simulink model "PMSM_SquareWave"  (R2021b)
settings: Solver=VariableStepAuto  StartTime=0.0  StopTime=500e-6  MaxStep=5e-8  RelTol=1e-5
InitFcn:
  | % Loading the measurement data
  | load('MeasurementData.mat', 'PM')
libraries: SLNS x2, simulink x2, simulink_extras x1
settings Model: Creator=Szalay  LastModifiedBy=Szalay
settings SolverCC: AlgebraicLoopSolver=TrustRegion
settings DebuggingCC: SFMachineParentedDataDiag=warning

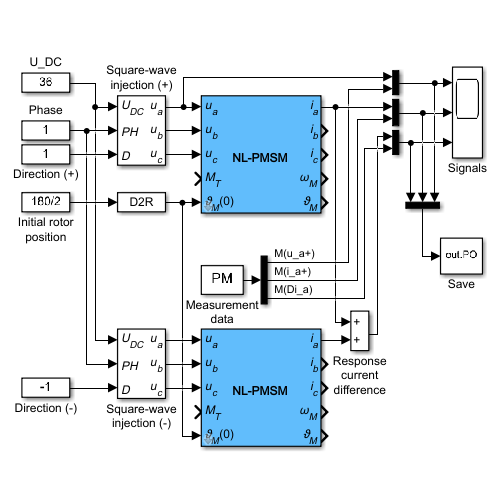
[thumbnail: Simulink's stored preview of the top-level diagram]
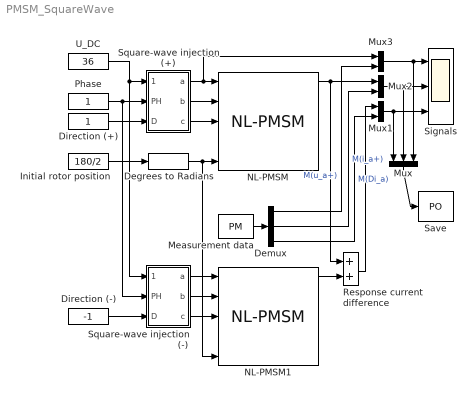
== system PMSM_SquareWave ==
  Degrees to Radians : simulink_extras/Transformations/Degrees to Radians
  Demux : Demux  Outputs=3
  Direction (+) : Constant
  Direction (-) : Constant  Value=-1
  Initial rotor position : Constant  Value=180/2
  Measurement data : FromWorkspace  VariableName=PM  SampleTime=-1  Interpolate=off  OutputAfterFinalValue=Setting to zero
  Mux : Mux  Inputs=3
  Mux1 : Mux  Inputs=2
  Mux2 : Mux  Inputs=2
  Mux3 : Mux  Inputs=2
  NL-PMSM : SLNS/Electric machines/NL-PMSM  varZp=2  varRs=0.654  varF_PM=24.83  varLd=145  varLq=188  varG_0=0.16  varB=6.329e-3  varJ=200  i_d0=0  i_q0=0
  NL-PMSM1 : SLNS/Electric machines/NL-PMSM  varZp=2  varRs=0.654  varF_PM=24.83  varLd=145  varLq=188  varG_0=0.16  varB=6.329e-3  varJ=200  i_d0=0  i_q0=0
  Phase : Constant
  Response current difference : Sum
  Save : ToWorkspace  VariableName=PO  SampleTime=1/240000
  Signals : Scope  NumInputPorts=3
  Square-wave injection (+) : Subsystem
      mask Display:
      | port_label('input', 1, '\itU_{DC}', 'texmode', 'on');
      | port_label('input', 2, '\itPH', 'texmode', 'on');
      | port_label('input', 3, '\itD', 'texmode', 'on');
      | 
      | port_label('output', 1, '\itu_a', 'texmode', 'on');
      | port_label('output', 2, '\itu_b', 'texmode', 'on');
      | port_label('output', 3, '\itu_c', 'texmode', 'on');
  Square-wave injection (-) : Subsystem
      mask Display:
      | port_label('input', 1, '\itU_{DC}', 'texmode', 'on');
      | port_label('input', 2, '\itPH', 'texmode', 'on');
      | port_label('input', 3, '\itD', 'texmode', 'on');
      | 
      | port_label('output', 1, '\itu_a', 'texmode', 'on');
      | port_label('output', 2, '\itu_b', 'texmode', 'on');
      | port_label('output', 3, '\itu_c', 'texmode', 'on');
  U_DC : Constant  Value=36
  wires:
  Initial rotor position/1 -> Degrees to Radians/1
  Square-wave injection (+)/1(a) -> NL-PMSM/1, Mux3/1
  Square-wave injection (+)/2(b) -> NL-PMSM/2
  Measurement data/1 -> Demux/1
  Demux/3 -> Mux1/2  "M(Di_a)"
  Demux/2 -> Mux2/2  "M(i_a+)"
  Demux/1 -> Mux3/2  "M(u_a+)"
  Response current difference/1 -> Mux1/1
  Square-wave injection (+)/3(c) -> NL-PMSM/3
  Direction (+)/1 -> Square-wave injection (+)/3(D)
  NL-PMSM/1 -> Mux2/1, Response current difference/1
  Direction (-)/1 -> Square-wave injection (-)/3(D)
  Phase/1 -> Square-wave injection (-)/2(PH), Square-wave injection (+)/2(PH)
  Square-wave injection (-)/3(c) -> NL-PMSM1/3
  Square-wave injection (-)/2(b) -> NL-PMSM1/2
  Square-wave injection (-)/1(a) -> NL-PMSM1/1
  Degrees to Radians/1 -> NL-PMSM1/5, NL-PMSM/5
  U_DC/1 -> Square-wave injection (-)/1(U_DC), Square-wave injection (+)/1(U_DC)
  NL-PMSM1/1 -> Response current difference/2
  Mux/1 -> Save/1
  Mux2/1 -> Mux/2, Signals/2
  Mux1/1 -> Mux/1, Signals/3
  Mux3/1 -> Mux/3, Signals/1

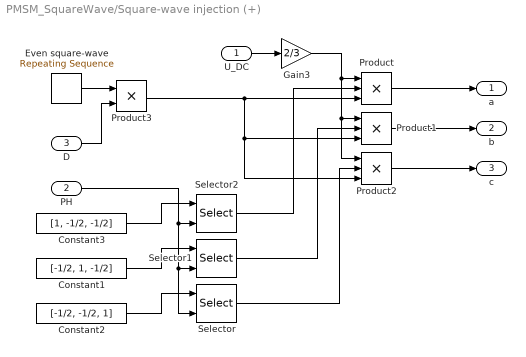
== system PMSM_SquareWave/Square-wave injection (+) ==
  U_DC : Inport
  PH : Inport  Port=2
  D : Inport  Port=3
  Constant1 : Constant  Value=[-1/2, 1, -1/2]
  Constant2 : Constant  Value=[-1/2, -1/2, 1]
  Constant3 : Constant  Value=[1, -1/2, -1/2]
  Even square-wave : simulink/Sources/Repeating Sequence  rep_seq_t=[0 1 1.05 2 2.05 4 4.05 5 5.05 2500]*75e-6  rep_seq_y="[0 0 1     1 -1    -1 1     1 0     0]"
  Gain3 : Gain  Gain=2/3
  Product : Product  Inputs=3
  Product1 : Product  Inputs=3
  Product2 : Product  Inputs=3
  Product3 : Product
  Selector : Selector  InputPortWidth=3  IndexOptions=Index vector (port)  Indices=[1 3]  OutputSizes=1
  Selector1 : Selector  InputPortWidth=3  IndexOptions=Index vector (port)  Indices=[1 3]  OutputSizes=1
  Selector2 : Selector  InputPortWidth=3  IndexOptions=Index vector (port)  Indices=[1 3]  OutputSizes=1
  a : Outport
  b : Outport  Port=2
  c : Outport  Port=3
  wires:
  Gain3/1 -> Product/1, Product2/1, Product1/1
  Even square-wave/1 -> Product3/1
  D/1 -> Product3/2
  U_DC/1 -> Gain3/1
  Product1/1 -> b/1
  Product2/1 -> c/1
  Product/1 -> a/1
  Product3/1 -> Product2/3, Product1/3, Product/3
  Selector2/1 -> Product/2
  Selector1/1 -> Product1/2
  Selector/1 -> Product2/2
  Constant3/1 -> Selector2/1
  Constant1/1 -> Selector1/1
  Constant2/1 -> Selector/1
  PH/1 -> Selector2/2, Selector1/2, Selector/2

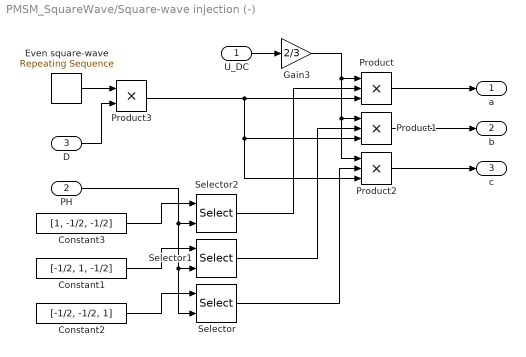
== system PMSM_SquareWave/Square-wave injection (-) ==
  U_DC : Inport
  PH : Inport  Port=2
  D : Inport  Port=3
  Constant1 : Constant  Value=[-1/2, 1, -1/2]
  Constant2 : Constant  Value=[-1/2, -1/2, 1]
  Constant3 : Constant  Value=[1, -1/2, -1/2]
  Even square-wave : simulink/Sources/Repeating Sequence  rep_seq_t=[0 1 1.05 2 2.05 4 4.05 5 5.05 2500]*75e-6  rep_seq_y="[0 0 1     1 -1    -1 1     1 0     0]"
  Gain3 : Gain  Gain=2/3
  Product : Product  Inputs=3
  Product1 : Product  Inputs=3
  Product2 : Product  Inputs=3
  Product3 : Product
  Selector : Selector  InputPortWidth=3  IndexOptions=Index vector (port)  Indices=[1 3]  OutputSizes=1
  Selector1 : Selector  InputPortWidth=3  IndexOptions=Index vector (port)  Indices=[1 3]  OutputSizes=1
  Selector2 : Selector  InputPortWidth=3  IndexOptions=Index vector (port)  Indices=[1 3]  OutputSizes=1
  a : Outport
  b : Outport  Port=2
  c : Outport  Port=3
  wires:
  PH/1 -> Selector/2, Selector1/2, Selector2/2
  Constant2/1 -> Selector/1
  Constant1/1 -> Selector1/1
  Constant3/1 -> Selector2/1
  Selector/1 -> Product2/2
  Selector1/1 -> Product1/2
  Selector2/1 -> Product/2
  Product3/1 -> Product/3, Product1/3, Product2/3
  Product/1 -> a/1
  Product2/1 -> c/1
  Product1/1 -> b/1
  U_DC/1 -> Gain3/1
  D/1 -> Product3/2
  Even square-wave/1 -> Product3/1
  Gain3/1 -> Product1/1, Product2/1, Product/1
